simulink model "modell_v3"  (Simulink 10.1)
settings: Solver=FixedStepAuto  StartTime=0.0  StopTime=10  FixedStep=1  RelTol=1e-3
settings Model: Creator=Bennu  LastModifiedBy=Piotr
settings DebuggingCC: UnderspecifiedInitializationDetection=Simplified  MergeDetectMultiDrivingBlocksExec=error  SFUnexpectedBacktrackingDiag=error  SFNoUnconditionalDefaultTransitionDiag=error
settings HardwareCC: ProdBitPerPointer=64  ProdLargestAtomicFloat=Float  ProdIntDivRoundTo=Zero  ProdEndianess=LittleEndian  ProdHWDeviceType=Specified
settings ModelReferenceCC: PropagateSignalLabelsOutOfModel=on
settings SFSimCC: SimUseLocalCustomCode=on
settings RTWCC: RTWUseLocalCustomCode=on
settings GRTTargetCC: TargetLangStandard=C99 (ISO)  CombineOutputUpdateFcns=on  GRTInterface=off
settings ConfigComp: CovMetricSettings=dwe  CovHtmlReporting=off  CovSaveCumulativeToWorkspaceVar=off  CovSaveSingleToWorkspaceVar=off  CovExternalEMLEnable=on

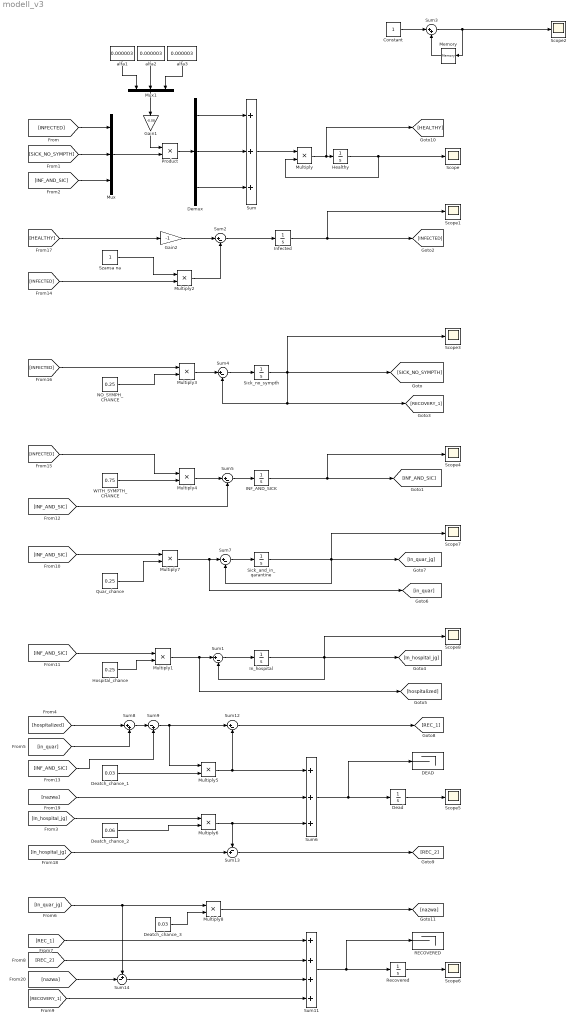
== system modell_v3 ==
  Constant : Constant
  DEAD : Terminator
  Dead : Integrator
  Deatch_chance_1 : Constant  Value=0.03
  Deatch_chance_2 : Constant  Value=0.06
  Deatch_chance_3 : Constant  Value=0.03
  Demux : Demux  Outputs=3
  Gain1 : Gain  Gain=-0.08
  Gain2 : Gain  Gain=-1
  Healthy : Integrator  InitialCondition=3000000
  Hospital_chance : Constant  Value=0.25
  INF_AND_SICK : Integrator  LowerSaturationLimit=0
  In_hospital : Integrator
  Infected : Integrator  InitialCondition=1  LowerSaturationLimit=0
  Memory : Memory
  Multiply{,1..8} (9 alike) : Product
  Mux : Mux  Inputs=3
  Mux1 : Mux  Inputs=3
  NO_SYMPH_CHANCE : Constant  Value=0.25
  Product : Product
  Quar_chance : Constant  Value=0.25
  RECOVERED : Terminator
  Recovered : Integrator
  Scope{,1..8} (9 alike) : Scope
  Sick_and_in_qarantine : Integrator
  Sick_no_sympth : Integrator  LowerSaturationLimit=0
  Sum : Sum  Inputs=+++
  Sum{1..2,4..5,7,12} (6 alike) : Sum  Inputs=|+-
  Sum11 : Sum  Inputs=++++
  Sum13 : Sum  Inputs=-+|
  Sum14 : Sum  Inputs=+-|
  Sum3 : Sum  Inputs=|++
  Sum6 : Sum  Inputs=+++
  Sum8 : Sum  Inputs=|++
  Sum9 : Sum  Inputs=|-+
  Szansa na : Constant
  WITH_SYMPTH_CHANCE : Constant  Value=0.75
  alfa1 : Constant  Value=0.000003
  alfa2 : Constant  Value=0.000003
  alfa3 : Constant  Value=0.000003
  wires:
  Multiply3/1 -> Sum4/1
  [INFECTED] -> Mux/1
  [SICK_NO_SYMPTH] -> Mux/2
  [INF_AND_SIC] -> Mux/3
  Multiply/1 -> [HEALTHY], Healthy/1
  Gain2/1 -> Sum2/1
  Szansa na/1 -> Multiply2/1
  Sum2/1 -> Infected/1
  NO_SYMPH_CHANCE/1 -> Multiply3/2
  Multiply4/1 -> Sum5/1
  WITH_SYMPTH_CHANCE/1 -> Multiply4/2
  Constant/1 -> Sum3/1
  Memory/1 -> Sum3/2
  Sum3/1 -> Scope2/1, Memory/1
  Multiply2/1 -> Sum2/2
  Infected/1 -> [INFECTED], Scope1/1
  Sum4/1 -> Sick_no_sympth/1
  Sick_no_sympth/1 -> Scope3/1, [SICK_NO_SYMPTH], Sum4/2, [RECOVERY_1]
  Sum5/1 -> INF_AND_SICK/1
  Hospital_chance/1 -> Multiply1/2
  Multiply1/1 -> Sum1/1, [hospitalized]
  Sum1/1 -> In_hospital/1
  In_hospital/1 -> Sum1/2, Scope8/1, [In_hospital_jg]
  Deatch_chance_1/1 -> Multiply5/2
  Multiply5/1 -> Sum6/1, Sum12/2
  Sum6/1 -> DEAD/1, Dead/1
  [In_hospital_jg] -> Multiply6/1
  Deatch_chance_2/1 -> Multiply6/2
  Multiply6/1 -> Sum13/1, Sum6/3
  Quar_chance/1 -> Multiply7/2
  Sum7/1 -> Sick_and_in_qarantine/1
  Multiply7/1 -> Sum7/1, [in_quar]
  INF_AND_SICK/1 -> Scope4/1, [INF_AND_SIC]
  Sum9/1 -> Sum12/1, Multiply5/1
  [hospitalized] -> Sum8/1
  [in_quar] -> Sum8/2
  Sum8/1 -> Sum9/1
  Dead/1 -> Scope5/1
  Sick_and_in_qarantine/1 -> Scope7/1, Sum7/2, [In_quar_jg]
  Deatch_chance_3/1 -> Multiply8/2
  [In_quar_jg] -> Sum14/1, Multiply8/1
  Sum11/1 -> RECOVERED/1, Recovered/1
  Sum12/1 -> [REC_1]
  [REC_1] -> Sum11/1
  Sum13/1 -> [REC_2]
  [REC_2] -> Sum11/2
  Sum14/1 -> Sum11/3
  Recovered/1 -> Scope6/1
  [RECOVERY_1] -> Sum11/4
  [INF_AND_SIC] -> Multiply7/1
  [INF_AND_SIC] -> Multiply1/1
  [INF_AND_SIC] -> Sum5/2
  [INF_AND_SIC] -> Sum9/2
  [INFECTED] -> Multiply2/2
  [INFECTED] -> Multiply4/1
  [INFECTED] -> Multiply3/1
  [HEALTHY] -> Gain2/1
  [In_hospital_jg] -> Sum13/2
  Multiply8/1 -> [nazwa]
  [nazwa] -> Sum6/2
  [nazwa] -> Sum14/2
  alfa1/1 -> Mux1/1
  alfa2/1 -> Mux1/2
  alfa3/1 -> Mux1/3
  Mux/1 -> Product/2
  Mux1/1 -> Gain1/1
  Gain1/1 -> Product/1
  Product/1 -> Demux/1
  Demux/1 -> Sum/1
  Demux/2 -> Sum/2
  Demux/3 -> Sum/3
  Sum/1 -> Multiply/1
  Healthy/1 -> Multiply/2, Scope/1
